simulink model "labFinal_8"  (R2018b)
settings: Solver=FixedStepDiscrete  StartTime=0.0  StopTime=20.0  FixedStep=1  RelTol=1e-3
libraries: hdlsllib x113, simulink_extras x8
(part 3 of 4)

== system labFinal_8/8-Bit_Processor/8-bit 4-1 MUX/4-1 MUX 2^6/2-1 MUX1 ==
  S : Inport  OutDataTypeStr=boolean
  I0 : Inport  Port=2  OutDataTypeStr=boolean
  I1 : Inport  Port=3  OutDataTypeStr=boolean
  Logical Operator : Logic  AllPortsSameDT=off  OutDataTypeStr=boolean
  Logical Operator1 : Logic  AllPortsSameDT=off  OutDataTypeStr=boolean
  Logical Operator2 : Logic  Operator=OR  AllPortsSameDT=off  OutDataTypeStr=boolean
  Logical Operator3 : Logic  Operator=NOT  AllPortsSameDT=off  OutDataTypeStr=boolean
  Z : Outport
  wires:
  Logical Operator2/1 -> Z/1
  Logical Operator1/1 -> Logical Operator2/2
  S/1 -> Logical Operator3/1, Logical Operator1/1
  Logical Operator/1 -> Logical Operator2/1
  I0/1 -> Logical Operator/1
  I1/1 -> Logical Operator1/2
  Logical Operator3/1 -> Logical Operator/2

== system labFinal_8/8-Bit_Processor/8-bit 4-1 MUX/4-1 MUX 2^6/2-1 MUX2 ==
  S : Inport  OutDataTypeStr=boolean
  I0 : Inport  Port=2  OutDataTypeStr=boolean
  I1 : Inport  Port=3  OutDataTypeStr=boolean
  Logical Operator : Logic  AllPortsSameDT=off  OutDataTypeStr=boolean
  Logical Operator1 : Logic  AllPortsSameDT=off  OutDataTypeStr=boolean
  Logical Operator2 : Logic  Operator=OR  AllPortsSameDT=off  OutDataTypeStr=boolean
  Logical Operator3 : Logic  Operator=NOT  AllPortsSameDT=off  OutDataTypeStr=boolean
  Z : Outport
  wires:
  Logical Operator2/1 -> Z/1
  Logical Operator1/1 -> Logical Operator2/2
  S/1 -> Logical Operator3/1, Logical Operator1/1
  Logical Operator/1 -> Logical Operator2/1
  I0/1 -> Logical Operator/1
  I1/1 -> Logical Operator1/2
  Logical Operator3/1 -> Logical Operator/2

== system labFinal_8/8-Bit_Processor/8-bit 4-1 MUX/4-1 MUX 2^6/2-1 MUX3 ==
  S : Inport  OutDataTypeStr=boolean
  I0 : Inport  Port=2  OutDataTypeStr=boolean
  I1 : Inport  Port=3  OutDataTypeStr=boolean
  Logical Operator : Logic  AllPortsSameDT=off  OutDataTypeStr=boolean
  Logical Operator1 : Logic  AllPortsSameDT=off  OutDataTypeStr=boolean
  Logical Operator2 : Logic  Operator=OR  AllPortsSameDT=off  OutDataTypeStr=boolean
  Logical Operator3 : Logic  Operator=NOT  AllPortsSameDT=off  OutDataTypeStr=boolean
  Z : Outport
  wires:
  Logical Operator2/1 -> Z/1
  Logical Operator1/1 -> Logical Operator2/2
  S/1 -> Logical Operator3/1, Logical Operator1/1
  Logical Operator/1 -> Logical Operator2/1
  I0/1 -> Logical Operator/1
  I1/1 -> Logical Operator1/2
  Logical Operator3/1 -> Logical Operator/2

== system labFinal_8/8-Bit_Processor/8-bit 4-1 MUX/4-1 MUX 2^7/2-1 MUX1 ==
  S : Inport  OutDataTypeStr=boolean
  I0 : Inport  Port=2  OutDataTypeStr=boolean
  I1 : Inport  Port=3  OutDataTypeStr=boolean
  Logical Operator : Logic  AllPortsSameDT=off  OutDataTypeStr=boolean
  Logical Operator1 : Logic  AllPortsSameDT=off  OutDataTypeStr=boolean
  Logical Operator2 : Logic  Operator=OR  AllPortsSameDT=off  OutDataTypeStr=boolean
  Logical Operator3 : Logic  Operator=NOT  AllPortsSameDT=off  OutDataTypeStr=boolean
  Z : Outport
  wires:
  Logical Operator2/1 -> Z/1
  Logical Operator1/1 -> Logical Operator2/2
  S/1 -> Logical Operator3/1, Logical Operator1/1
  Logical Operator/1 -> Logical Operator2/1
  I0/1 -> Logical Operator/1
  I1/1 -> Logical Operator1/2
  Logical Operator3/1 -> Logical Operator/2

== system labFinal_8/8-Bit_Processor/8-bit 4-1 MUX/4-1 MUX 2^7/2-1 MUX2 ==
  S : Inport  OutDataTypeStr=boolean
  I0 : Inport  Port=2  OutDataTypeStr=boolean
  I1 : Inport  Port=3  OutDataTypeStr=boolean
  Logical Operator : Logic  AllPortsSameDT=off  OutDataTypeStr=boolean
  Logical Operator1 : Logic  AllPortsSameDT=off  OutDataTypeStr=boolean
  Logical Operator2 : Logic  Operator=OR  AllPortsSameDT=off  OutDataTypeStr=boolean
  Logical Operator3 : Logic  Operator=NOT  AllPortsSameDT=off  OutDataTypeStr=boolean
  Z : Outport
  wires:
  Logical Operator2/1 -> Z/1
  Logical Operator1/1 -> Logical Operator2/2
  S/1 -> Logical Operator3/1, Logical Operator1/1
  Logical Operator/1 -> Logical Operator2/1
  I0/1 -> Logical Operator/1
  I1/1 -> Logical Operator1/2
  Logical Operator3/1 -> Logical Operator/2

== system labFinal_8/8-Bit_Processor/8-bit 4-1 MUX/4-1 MUX 2^7/2-1 MUX3 ==
  S : Inport  OutDataTypeStr=boolean
  I0 : Inport  Port=2  OutDataTypeStr=boolean
  I1 : Inport  Port=3  OutDataTypeStr=boolean
  Logical Operator : Logic  AllPortsSameDT=off  OutDataTypeStr=boolean
  Logical Operator1 : Logic  AllPortsSameDT=off  OutDataTypeStr=boolean
  Logical Operator2 : Logic  Operator=OR  AllPortsSameDT=off  OutDataTypeStr=boolean
  Logical Operator3 : Logic  Operator=NOT  AllPortsSameDT=off  OutDataTypeStr=boolean
  Z : Outport
  wires:
  Logical Operator2/1 -> Z/1
  Logical Operator1/1 -> Logical Operator2/2
  S/1 -> Logical Operator3/1, Logical Operator1/1
  Logical Operator/1 -> Logical Operator2/1
  I0/1 -> Logical Operator/1
  I1/1 -> Logical Operator1/2
  Logical Operator3/1 -> Logical Operator/2

== system labFinal_8/8-Bit_Processor/8-bit 4-1 MUX/4-1 MUX 2^8/2-1 MUX1 ==
  S : Inport  OutDataTypeStr=boolean
  I0 : Inport  Port=2  OutDataTypeStr=boolean
  I1 : Inport  Port=3  OutDataTypeStr=boolean
  Logical Operator : Logic  AllPortsSameDT=off  OutDataTypeStr=boolean
  Logical Operator1 : Logic  AllPortsSameDT=off  OutDataTypeStr=boolean
  Logical Operator2 : Logic  Operator=OR  AllPortsSameDT=off  OutDataTypeStr=boolean
  Logical Operator3 : Logic  Operator=NOT  AllPortsSameDT=off  OutDataTypeStr=boolean
  Z : Outport
  wires:
  Logical Operator2/1 -> Z/1
  Logical Operator1/1 -> Logical Operator2/2
  S/1 -> Logical Operator3/1, Logical Operator1/1
  Logical Operator/1 -> Logical Operator2/1
  I0/1 -> Logical Operator/1
  I1/1 -> Logical Operator1/2
  Logical Operator3/1 -> Logical Operator/2

== system labFinal_8/8-Bit_Processor/8-bit 4-1 MUX/4-1 MUX 2^8/2-1 MUX2 ==
  S : Inport  OutDataTypeStr=boolean
  I0 : Inport  Port=2  OutDataTypeStr=boolean
  I1 : Inport  Port=3  OutDataTypeStr=boolean
  Logical Operator : Logic  AllPortsSameDT=off  OutDataTypeStr=boolean
  Logical Operator1 : Logic  AllPortsSameDT=off  OutDataTypeStr=boolean
  Logical Operator2 : Logic  Operator=OR  AllPortsSameDT=off  OutDataTypeStr=boolean
  Logical Operator3 : Logic  Operator=NOT  AllPortsSameDT=off  OutDataTypeStr=boolean
  Z : Outport
  wires:
  Logical Operator2/1 -> Z/1
  Logical Operator1/1 -> Logical Operator2/2
  S/1 -> Logical Operator3/1, Logical Operator1/1
  Logical Operator/1 -> Logical Operator2/1
  I0/1 -> Logical Operator/1
  I1/1 -> Logical Operator1/2
  Logical Operator3/1 -> Logical Operator/2

== system labFinal_8/8-Bit_Processor/8-bit 4-1 MUX/4-1 MUX 2^8/2-1 MUX3 ==
  S : Inport  OutDataTypeStr=boolean
  I0 : Inport  Port=2  OutDataTypeStr=boolean
  I1 : Inport  Port=3  OutDataTypeStr=boolean
  Logical Operator : Logic  AllPortsSameDT=off  OutDataTypeStr=boolean
  Logical Operator1 : Logic  AllPortsSameDT=off  OutDataTypeStr=boolean
  Logical Operator2 : Logic  Operator=OR  AllPortsSameDT=off  OutDataTypeStr=boolean
  Logical Operator3 : Logic  Operator=NOT  AllPortsSameDT=off  OutDataTypeStr=boolean
  Z : Outport
  wires:
  Logical Operator2/1 -> Z/1
  Logical Operator1/1 -> Logical Operator2/2
  S/1 -> Logical Operator3/1, Logical Operator1/1
  Logical Operator/1 -> Logical Operator2/1
  I0/1 -> Logical Operator/1
  I1/1 -> Logical Operator1/2
  Logical Operator3/1 -> Logical Operator/2

== system labFinal_8/8-Bit_Processor/8-bit Adder/2^0/Half_Adder ==
  x : Inport
  y : Inport  Port=2
  Calc Carry : Logic  AllPortsSameDT=off  OutDataTypeStr=boolean
  Calc Sum : Logic  Operator=XOR  AllPortsSameDT=off  OutDataTypeStr=boolean
  Sum : Outport
  Carry : Outport  Port=2
  wires:
  Calc Carry/1 -> Carry/1
  x/1 -> Calc Carry/1, Calc Sum/1
  Calc Sum/1 -> Sum/1
  y/1 -> Calc Sum/2, Calc Carry/2

== system labFinal_8/8-Bit_Processor/8-bit Adder/2^0/Half_Adder1 ==
  x : Inport
  y : Inport  Port=2
  Calc Carry : Logic  AllPortsSameDT=off  OutDataTypeStr=boolean
  Calc Sum : Logic  Operator=XOR  AllPortsSameDT=off  OutDataTypeStr=boolean
  Sum : Outport
  Carry : Outport  Port=2
  wires:
  Calc Carry/1 -> Carry/1
  x/1 -> Calc Carry/1, Calc Sum/1
  Calc Sum/1 -> Sum/1
  y/1 -> Calc Sum/2, Calc Carry/2

== system labFinal_8/8-Bit_Processor/8-bit Adder/2^1/Half_Adder ==
  x : Inport
  y : Inport  Port=2
  Calc Carry : Logic  AllPortsSameDT=off  OutDataTypeStr=boolean
  Calc Sum : Logic  Operator=XOR  AllPortsSameDT=off  OutDataTypeStr=boolean
  Sum : Outport
  Carry : Outport  Port=2
  wires:
  Calc Carry/1 -> Carry/1
  x/1 -> Calc Carry/1, Calc Sum/1
  Calc Sum/1 -> Sum/1
  y/1 -> Calc Sum/2, Calc Carry/2

== system labFinal_8/8-Bit_Processor/8-bit Adder/2^1/Half_Adder1 ==
  x : Inport
  y : Inport  Port=2
  Calc Carry : Logic  AllPortsSameDT=off  OutDataTypeStr=boolean
  Calc Sum : Logic  Operator=XOR  AllPortsSameDT=off  OutDataTypeStr=boolean
  Sum : Outport
  Carry : Outport  Port=2
  wires:
  Calc Carry/1 -> Carry/1
  x/1 -> Calc Carry/1, Calc Sum/1
  Calc Sum/1 -> Sum/1
  y/1 -> Calc Sum/2, Calc Carry/2

== system labFinal_8/8-Bit_Processor/8-bit Adder/2^2/Half_Adder ==
  x : Inport
  y : Inport  Port=2
  Calc Carry : Logic  AllPortsSameDT=off  OutDataTypeStr=boolean
  Calc Sum : Logic  Operator=XOR  AllPortsSameDT=off  OutDataTypeStr=boolean
  Sum : Outport
  Carry : Outport  Port=2
  wires:
  Calc Carry/1 -> Carry/1
  x/1 -> Calc Carry/1, Calc Sum/1
  Calc Sum/1 -> Sum/1
  y/1 -> Calc Sum/2, Calc Carry/2

== system labFinal_8/8-Bit_Processor/8-bit Adder/2^2/Half_Adder1 ==
  x : Inport
  y : Inport  Port=2
  Calc Carry : Logic  AllPortsSameDT=off  OutDataTypeStr=boolean
  Calc Sum : Logic  Operator=XOR  AllPortsSameDT=off  OutDataTypeStr=boolean
  Sum : Outport
  Carry : Outport  Port=2
  wires:
  Calc Carry/1 -> Carry/1
  x/1 -> Calc Carry/1, Calc Sum/1
  Calc Sum/1 -> Sum/1
  y/1 -> Calc Sum/2, Calc Carry/2

== system labFinal_8/8-Bit_Processor/8-bit Adder/2^3/Half_Adder ==
  x : Inport
  y : Inport  Port=2
  Calc Carry : Logic  AllPortsSameDT=off  OutDataTypeStr=boolean
  Calc Sum : Logic  Operator=XOR  AllPortsSameDT=off  OutDataTypeStr=boolean
  Sum : Outport
  Carry : Outport  Port=2
  wires:
  Calc Carry/1 -> Carry/1
  x/1 -> Calc Carry/1, Calc Sum/1
  Calc Sum/1 -> Sum/1
  y/1 -> Calc Sum/2, Calc Carry/2

== system labFinal_8/8-Bit_Processor/8-bit Adder/2^3/Half_Adder1 ==
  x : Inport
  y : Inport  Port=2
  Calc Carry : Logic  AllPortsSameDT=off  OutDataTypeStr=boolean
  Calc Sum : Logic  Operator=XOR  AllPortsSameDT=off  OutDataTypeStr=boolean
  Sum : Outport
  Carry : Outport  Port=2
  wires:
  Calc Carry/1 -> Carry/1
  x/1 -> Calc Carry/1, Calc Sum/1
  Calc Sum/1 -> Sum/1
  y/1 -> Calc Sum/2, Calc Carry/2

== system labFinal_8/8-Bit_Processor/8-bit Adder/2^4/Half_Adder ==
  x : Inport
  y : Inport  Port=2
  Calc Carry : Logic  AllPortsSameDT=off  OutDataTypeStr=boolean
  Calc Sum : Logic  Operator=XOR  AllPortsSameDT=off  OutDataTypeStr=boolean
  Sum : Outport
  Carry : Outport  Port=2
  wires:
  Calc Carry/1 -> Carry/1
  x/1 -> Calc Carry/1, Calc Sum/1
  Calc Sum/1 -> Sum/1
  y/1 -> Calc Sum/2, Calc Carry/2

== system labFinal_8/8-Bit_Processor/8-bit Adder/2^4/Half_Adder1 ==
  x : Inport
  y : Inport  Port=2
  Calc Carry : Logic  AllPortsSameDT=off  OutDataTypeStr=boolean
  Calc Sum : Logic  Operator=XOR  AllPortsSameDT=off  OutDataTypeStr=boolean
  Sum : Outport
  Carry : Outport  Port=2
  wires:
  Calc Carry/1 -> Carry/1
  x/1 -> Calc Carry/1, Calc Sum/1
  Calc Sum/1 -> Sum/1
  y/1 -> Calc Sum/2, Calc Carry/2

== system labFinal_8/8-Bit_Processor/8-bit Adder/2^5/Half_Adder ==
  x : Inport
  y : Inport  Port=2
  Calc Carry : Logic  AllPortsSameDT=off  OutDataTypeStr=boolean
  Calc Sum : Logic  Operator=XOR  AllPortsSameDT=off  OutDataTypeStr=boolean
  Sum : Outport
  Carry : Outport  Port=2
  wires:
  Calc Carry/1 -> Carry/1
  x/1 -> Calc Carry/1, Calc Sum/1
  Calc Sum/1 -> Sum/1
  y/1 -> Calc Sum/2, Calc Carry/2

== system labFinal_8/8-Bit_Processor/8-bit Adder/2^5/Half_Adder1 ==
  x : Inport
  y : Inport  Port=2
  Calc Carry : Logic  AllPortsSameDT=off  OutDataTypeStr=boolean
  Calc Sum : Logic  Operator=XOR  AllPortsSameDT=off  OutDataTypeStr=boolean
  Sum : Outport
  Carry : Outport  Port=2
  wires:
  Calc Carry/1 -> Carry/1
  x/1 -> Calc Carry/1, Calc Sum/1
  Calc Sum/1 -> Sum/1
  y/1 -> Calc Sum/2, Calc Carry/2

== system labFinal_8/8-Bit_Processor/8-bit Adder/2^6/Half_Adder ==
  x : Inport
  y : Inport  Port=2
  Calc Carry : Logic  AllPortsSameDT=off  OutDataTypeStr=boolean
  Calc Sum : Logic  Operator=XOR  AllPortsSameDT=off  OutDataTypeStr=boolean
  Sum : Outport
  Carry : Outport  Port=2
  wires:
  Calc Carry/1 -> Carry/1
  x/1 -> Calc Carry/1, Calc Sum/1
  Calc Sum/1 -> Sum/1
  y/1 -> Calc Sum/2, Calc Carry/2

== system labFinal_8/8-Bit_Processor/8-bit Adder/2^6/Half_Adder1 ==
  x : Inport
  y : Inport  Port=2
  Calc Carry : Logic  AllPortsSameDT=off  OutDataTypeStr=boolean
  Calc Sum : Logic  Operator=XOR  AllPortsSameDT=off  OutDataTypeStr=boolean
  Sum : Outport
  Carry : Outport  Port=2
  wires:
  Calc Carry/1 -> Carry/1
  x/1 -> Calc Carry/1, Calc Sum/1
  Calc Sum/1 -> Sum/1
  y/1 -> Calc Sum/2, Calc Carry/2

== system labFinal_8/8-Bit_Processor/8-bit Adder/2^7/Half_Adder ==
  x : Inport
  y : Inport  Port=2
  Calc Carry : Logic  AllPortsSameDT=off  OutDataTypeStr=boolean
  Calc Sum : Logic  Operator=XOR  AllPortsSameDT=off  OutDataTypeStr=boolean
  Sum : Outport
  Carry : Outport  Port=2
  wires:
  Calc Carry/1 -> Carry/1
  x/1 -> Calc Carry/1, Calc Sum/1
  Calc Sum/1 -> Sum/1
  y/1 -> Calc Sum/2, Calc Carry/2

== system labFinal_8/8-Bit_Processor/8-bit Adder/2^7/Half_Adder1 ==
  x : Inport
  y : Inport  Port=2
  Calc Carry : Logic  AllPortsSameDT=off  OutDataTypeStr=boolean
  Calc Sum : Logic  Operator=XOR  AllPortsSameDT=off  OutDataTypeStr=boolean
  Sum : Outport
  Carry : Outport  Port=2
  wires:
  Calc Carry/1 -> Carry/1
  x/1 -> Calc Carry/1, Calc Sum/1
  Calc Sum/1 -> Sum/1
  y/1 -> Calc Sum/2, Calc Carry/2

== system labFinal_8/8-Bit_Processor/8-bit Multiply/2^1/Half_Adder ==
  x : Inport
  y : Inport  Port=2
  Calc Carry : Logic  AllPortsSameDT=off  OutDataTypeStr=boolean
  Calc Sum : Logic  Operator=XOR  AllPortsSameDT=off  OutDataTypeStr=boolean
  Sum : Outport
  Carry : Outport  Port=2
  wires:
  Calc Carry/1 -> Carry/1
  x/1 -> Calc Carry/1, Calc Sum/1
  Calc Sum/1 -> Sum/1
  y/1 -> Calc Sum/2, Calc Carry/2

== system labFinal_8/8-Bit_Processor/8-bit Multiply/2^1/Half_Adder1 ==
  x : Inport
  y : Inport  Port=2
  Calc Carry : Logic  AllPortsSameDT=off  OutDataTypeStr=boolean
  Calc Sum : Logic  Operator=XOR  AllPortsSameDT=off  OutDataTypeStr=boolean
  Sum : Outport
  Carry : Outport  Port=2
  wires:
  Calc Carry/1 -> Carry/1
  x/1 -> Calc Carry/1, Calc Sum/1
  Calc Sum/1 -> Sum/1
  y/1 -> Calc Sum/2, Calc Carry/2

== system labFinal_8/8-Bit_Processor/8-bit Multiply/2^10/Half_Adder ==
  x : Inport
  y : Inport  Port=2
  Calc Carry : Logic  AllPortsSameDT=off  OutDataTypeStr=boolean
  Calc Sum : Logic  Operator=XOR  AllPortsSameDT=off  OutDataTypeStr=boolean
  Sum : Outport
  Carry : Outport  Port=2
  wires:
  Calc Carry/1 -> Carry/1
  x/1 -> Calc Carry/1, Calc Sum/1
  Calc Sum/1 -> Sum/1
  y/1 -> Calc Sum/2, Calc Carry/2

== system labFinal_8/8-Bit_Processor/8-bit Multiply/2^10/Half_Adder1 ==
  x : Inport
  y : Inport  Port=2
  Calc Carry : Logic  AllPortsSameDT=off  OutDataTypeStr=boolean
  Calc Sum : Logic  Operator=XOR  AllPortsSameDT=off  OutDataTypeStr=boolean
  Sum : Outport
  Carry : Outport  Port=2
  wires:
  Calc Carry/1 -> Carry/1
  x/1 -> Calc Carry/1, Calc Sum/1
  Calc Sum/1 -> Sum/1
  y/1 -> Calc Sum/2, Calc Carry/2

== system labFinal_8/8-Bit_Processor/8-bit Multiply/2^11/Half_Adder ==
  x : Inport
  y : Inport  Port=2
  Calc Carry : Logic  AllPortsSameDT=off  OutDataTypeStr=boolean
  Calc Sum : Logic  Operator=XOR  AllPortsSameDT=off  OutDataTypeStr=boolean
  Sum : Outport
  Carry : Outport  Port=2
  wires:
  Calc Carry/1 -> Carry/1
  x/1 -> Calc Carry/1, Calc Sum/1
  Calc Sum/1 -> Sum/1
  y/1 -> Calc Sum/2, Calc Carry/2

== system labFinal_8/8-Bit_Processor/8-bit Multiply/2^11/Half_Adder1 ==
  x : Inport
  y : Inport  Port=2
  Calc Carry : Logic  AllPortsSameDT=off  OutDataTypeStr=boolean
  Calc Sum : Logic  Operator=XOR  AllPortsSameDT=off  OutDataTypeStr=boolean
  Sum : Outport
  Carry : Outport  Port=2
  wires:
  Calc Carry/1 -> Carry/1
  x/1 -> Calc Carry/1, Calc Sum/1
  Calc Sum/1 -> Sum/1
  y/1 -> Calc Sum/2, Calc Carry/2

== system labFinal_8/8-Bit_Processor/8-bit Multiply/2^12/Half_Adder ==
  x : Inport
  y : Inport  Port=2
  Calc Carry : Logic  AllPortsSameDT=off  OutDataTypeStr=boolean
  Calc Sum : Logic  Operator=XOR  AllPortsSameDT=off  OutDataTypeStr=boolean
  Sum : Outport
  Carry : Outport  Port=2
  wires:
  Calc Carry/1 -> Carry/1
  x/1 -> Calc Carry/1, Calc Sum/1
  Calc Sum/1 -> Sum/1
  y/1 -> Calc Sum/2, Calc Carry/2

== system labFinal_8/8-Bit_Processor/8-bit Multiply/2^12/Half_Adder1 ==
  x : Inport
  y : Inport  Port=2
  Calc Carry : Logic  AllPortsSameDT=off  OutDataTypeStr=boolean
  Calc Sum : Logic  Operator=XOR  AllPortsSameDT=off  OutDataTypeStr=boolean
  Sum : Outport
  Carry : Outport  Port=2
  wires:
  Calc Carry/1 -> Carry/1
  x/1 -> Calc Carry/1, Calc Sum/1
  Calc Sum/1 -> Sum/1
  y/1 -> Calc Sum/2, Calc Carry/2

== system labFinal_8/8-Bit_Processor/8-bit Multiply/2^13/Half_Adder ==
  x : Inport
  y : Inport  Port=2
  Calc Carry : Logic  AllPortsSameDT=off  OutDataTypeStr=boolean
  Calc Sum : Logic  Operator=XOR  AllPortsSameDT=off  OutDataTypeStr=boolean
  Sum : Outport
  Carry : Outport  Port=2
  wires:
  Calc Carry/1 -> Carry/1
  x/1 -> Calc Carry/1, Calc Sum/1
  Calc Sum/1 -> Sum/1
  y/1 -> Calc Sum/2, Calc Carry/2

== system labFinal_8/8-Bit_Processor/8-bit Multiply/2^13/Half_Adder1 ==
  x : Inport
  y : Inport  Port=2
  Calc Carry : Logic  AllPortsSameDT=off  OutDataTypeStr=boolean
  Calc Sum : Logic  Operator=XOR  AllPortsSameDT=off  OutDataTypeStr=boolean
  Sum : Outport
  Carry : Outport  Port=2
  wires:
  Calc Carry/1 -> Carry/1
  x/1 -> Calc Carry/1, Calc Sum/1
  Calc Sum/1 -> Sum/1
  y/1 -> Calc Sum/2, Calc Carry/2

== system labFinal_8/8-Bit_Processor/8-bit Multiply/2^14/Half_Adder ==
  x : Inport
  y : Inport  Port=2
  Calc Carry : Logic  AllPortsSameDT=off  OutDataTypeStr=boolean
  Calc Sum : Logic  Operator=XOR  AllPortsSameDT=off  OutDataTypeStr=boolean
  Sum : Outport
  Carry : Outport  Port=2
  wires:
  Calc Carry/1 -> Carry/1
  x/1 -> Calc Carry/1, Calc Sum/1
  Calc Sum/1 -> Sum/1
  y/1 -> Calc Sum/2, Calc Carry/2

== system labFinal_8/8-Bit_Processor/8-bit Multiply/2^14/Half_Adder1 ==
  x : Inport
  y : Inport  Port=2
  Calc Carry : Logic  AllPortsSameDT=off  OutDataTypeStr=boolean
  Calc Sum : Logic  Operator=XOR  AllPortsSameDT=off  OutDataTypeStr=boolean
  Sum : Outport
  Carry : Outport  Port=2
  wires:
  Calc Carry/1 -> Carry/1
  x/1 -> Calc Carry/1, Calc Sum/1
  Calc Sum/1 -> Sum/1
  y/1 -> Calc Sum/2, Calc Carry/2

== system labFinal_8/8-Bit_Processor/8-bit Multiply/2^15/Half_Adder ==
  x : Inport
  y : Inport  Port=2
  Calc Carry : Logic  AllPortsSameDT=off  OutDataTypeStr=boolean
  Calc Sum : Logic  Operator=XOR  AllPortsSameDT=off  OutDataTypeStr=boolean
  Sum : Outport
  Carry : Outport  Port=2
  wires:
  Calc Carry/1 -> Carry/1
  x/1 -> Calc Carry/1, Calc Sum/1
  Calc Sum/1 -> Sum/1
  y/1 -> Calc Sum/2, Calc Carry/2

== system labFinal_8/8-Bit_Processor/8-bit Multiply/2^15/Half_Adder1 ==
  x : Inport
  y : Inport  Port=2
  Calc Carry : Logic  AllPortsSameDT=off  OutDataTypeStr=boolean
  Calc Sum : Logic  Operator=XOR  AllPortsSameDT=off  OutDataTypeStr=boolean
  Sum : Outport
  Carry : Outport  Port=2
  wires:
  Calc Carry/1 -> Carry/1
  x/1 -> Calc Carry/1, Calc Sum/1
  Calc Sum/1 -> Sum/1
  y/1 -> Calc Sum/2, Calc Carry/2

== system labFinal_8/8-Bit_Processor/8-bit Multiply/2^16/Half_Adder ==
  x : Inport
  y : Inport  Port=2
  Calc Carry : Logic  AllPortsSameDT=off  OutDataTypeStr=boolean
  Calc Sum : Logic  Operator=XOR  AllPortsSameDT=off  OutDataTypeStr=boolean
  Sum : Outport
  Carry : Outport  Port=2
  wires:
  Calc Carry/1 -> Carry/1
  x/1 -> Calc Carry/1, Calc Sum/1
  Calc Sum/1 -> Sum/1
  y/1 -> Calc Sum/2, Calc Carry/2

== system labFinal_8/8-Bit_Processor/8-bit Multiply/2^16/Half_Adder1 ==
  x : Inport
  y : Inport  Port=2
  Calc Carry : Logic  AllPortsSameDT=off  OutDataTypeStr=boolean
  Calc Sum : Logic  Operator=XOR  AllPortsSameDT=off  OutDataTypeStr=boolean
  Sum : Outport
  Carry : Outport  Port=2
  wires:
  Calc Carry/1 -> Carry/1
  x/1 -> Calc Carry/1, Calc Sum/1
  Calc Sum/1 -> Sum/1
  y/1 -> Calc Sum/2, Calc Carry/2

== system labFinal_8/8-Bit_Processor/8-bit Multiply/2^17/Half_Adder ==
  x : Inport
  y : Inport  Port=2
  Calc Carry : Logic  AllPortsSameDT=off  OutDataTypeStr=boolean
  Calc Sum : Logic  Operator=XOR  AllPortsSameDT=off  OutDataTypeStr=boolean
  Sum : Outport
  Carry : Outport  Port=2
  wires:
  Calc Carry/1 -> Carry/1
  x/1 -> Calc Carry/1, Calc Sum/1
  Calc Sum/1 -> Sum/1
  y/1 -> Calc Sum/2, Calc Carry/2

== system labFinal_8/8-Bit_Processor/8-bit Multiply/2^17/Half_Adder1 ==
  x : Inport
  y : Inport  Port=2
  Calc Carry : Logic  AllPortsSameDT=off  OutDataTypeStr=boolean
  Calc Sum : Logic  Operator=XOR  AllPortsSameDT=off  OutDataTypeStr=boolean
  Sum : Outport
  Carry : Outport  Port=2
  wires:
  Calc Carry/1 -> Carry/1
  x/1 -> Calc Carry/1, Calc Sum/1
  Calc Sum/1 -> Sum/1
  y/1 -> Calc Sum/2, Calc Carry/2

== system labFinal_8/8-Bit_Processor/8-bit Multiply/2^18/Half_Adder ==
  x : Inport
  y : Inport  Port=2
  Calc Carry : Logic  AllPortsSameDT=off  OutDataTypeStr=boolean
  Calc Sum : Logic  Operator=XOR  AllPortsSameDT=off  OutDataTypeStr=boolean
  Sum : Outport
  Carry : Outport  Port=2
  wires:
  Calc Carry/1 -> Carry/1
  x/1 -> Calc Carry/1, Calc Sum/1
  Calc Sum/1 -> Sum/1
  y/1 -> Calc Sum/2, Calc Carry/2

== system labFinal_8/8-Bit_Processor/8-bit Multiply/2^18/Half_Adder1 ==
  x : Inport
  y : Inport  Port=2
  Calc Carry : Logic  AllPortsSameDT=off  OutDataTypeStr=boolean
  Calc Sum : Logic  Operator=XOR  AllPortsSameDT=off  OutDataTypeStr=boolean
  Sum : Outport
  Carry : Outport  Port=2
  wires:
  Calc Carry/1 -> Carry/1
  x/1 -> Calc Carry/1, Calc Sum/1
  Calc Sum/1 -> Sum/1
  y/1 -> Calc Sum/2, Calc Carry/2

== system labFinal_8/8-Bit_Processor/8-bit Multiply/2^19/Half_Adder ==
  x : Inport
  y : Inport  Port=2
  Calc Carry : Logic  AllPortsSameDT=off  OutDataTypeStr=boolean
  Calc Sum : Logic  Operator=XOR  AllPortsSameDT=off  OutDataTypeStr=boolean
  Sum : Outport
  Carry : Outport  Port=2
  wires:
  Calc Carry/1 -> Carry/1
  x/1 -> Calc Carry/1, Calc Sum/1
  Calc Sum/1 -> Sum/1
  y/1 -> Calc Sum/2, Calc Carry/2

== system labFinal_8/8-Bit_Processor/8-bit Multiply/2^19/Half_Adder1 ==
  x : Inport
  y : Inport  Port=2
  Calc Carry : Logic  AllPortsSameDT=off  OutDataTypeStr=boolean
  Calc Sum : Logic  Operator=XOR  AllPortsSameDT=off  OutDataTypeStr=boolean
  Sum : Outport
  Carry : Outport  Port=2
  wires:
  Calc Carry/1 -> Carry/1
  x/1 -> Calc Carry/1, Calc Sum/1
  Calc Sum/1 -> Sum/1
  y/1 -> Calc Sum/2, Calc Carry/2

== system labFinal_8/8-Bit_Processor/8-bit Multiply/2^2/Half_Adder ==
  x : Inport
  y : Inport  Port=2
  Calc Carry : Logic  AllPortsSameDT=off  OutDataTypeStr=boolean
  Calc Sum : Logic  Operator=XOR  AllPortsSameDT=off  OutDataTypeStr=boolean
  Sum : Outport
  Carry : Outport  Port=2
  wires:
  Calc Carry/1 -> Carry/1
  x/1 -> Calc Carry/1, Calc Sum/1
  Calc Sum/1 -> Sum/1
  y/1 -> Calc Sum/2, Calc Carry/2

== system labFinal_8/8-Bit_Processor/8-bit Multiply/2^2/Half_Adder1 ==
  x : Inport
  y : Inport  Port=2
  Calc Carry : Logic  AllPortsSameDT=off  OutDataTypeStr=boolean
  Calc Sum : Logic  Operator=XOR  AllPortsSameDT=off  OutDataTypeStr=boolean
  Sum : Outport
  Carry : Outport  Port=2
  wires:
  Calc Carry/1 -> Carry/1
  x/1 -> Calc Carry/1, Calc Sum/1
  Calc Sum/1 -> Sum/1
  y/1 -> Calc Sum/2, Calc Carry/2

== system labFinal_8/8-Bit_Processor/8-bit Multiply/2^20/Half_Adder ==
  x : Inport
  y : Inport  Port=2
  Calc Carry : Logic  AllPortsSameDT=off  OutDataTypeStr=boolean
  Calc Sum : Logic  Operator=XOR  AllPortsSameDT=off  OutDataTypeStr=boolean
  Sum : Outport
  Carry : Outport  Port=2
  wires:
  Calc Carry/1 -> Carry/1
  x/1 -> Calc Carry/1, Calc Sum/1
  Calc Sum/1 -> Sum/1
  y/1 -> Calc Sum/2, Calc Carry/2

== system labFinal_8/8-Bit_Processor/8-bit Multiply/2^20/Half_Adder1 ==
  x : Inport
  y : Inport  Port=2
  Calc Carry : Logic  AllPortsSameDT=off  OutDataTypeStr=boolean
  Calc Sum : Logic  Operator=XOR  AllPortsSameDT=off  OutDataTypeStr=boolean
  Sum : Outport
  Carry : Outport  Port=2
  wires:
  Calc Carry/1 -> Carry/1
  x/1 -> Calc Carry/1, Calc Sum/1
  Calc Sum/1 -> Sum/1
  y/1 -> Calc Sum/2, Calc Carry/2

== system labFinal_8/8-Bit_Processor/8-bit Multiply/2^21/Half_Adder ==
  x : Inport
  y : Inport  Port=2
  Calc Carry : Logic  AllPortsSameDT=off  OutDataTypeStr=boolean
  Calc Sum : Logic  Operator=XOR  AllPortsSameDT=off  OutDataTypeStr=boolean
  Sum : Outport
  Carry : Outport  Port=2
  wires:
  Calc Carry/1 -> Carry/1
  x/1 -> Calc Carry/1, Calc Sum/1
  Calc Sum/1 -> Sum/1
  y/1 -> Calc Sum/2, Calc Carry/2

== system labFinal_8/8-Bit_Processor/8-bit Multiply/2^21/Half_Adder1 ==
  x : Inport
  y : Inport  Port=2
  Calc Carry : Logic  AllPortsSameDT=off  OutDataTypeStr=boolean
  Calc Sum : Logic  Operator=XOR  AllPortsSameDT=off  OutDataTypeStr=boolean
  Sum : Outport
  Carry : Outport  Port=2
  wires:
  Calc Carry/1 -> Carry/1
  x/1 -> Calc Carry/1, Calc Sum/1
  Calc Sum/1 -> Sum/1
  y/1 -> Calc Sum/2, Calc Carry/2

== system labFinal_8/8-Bit_Processor/8-bit Multiply/2^22/Half_Adder ==
  x : Inport
  y : Inport  Port=2
  Calc Carry : Logic  AllPortsSameDT=off  OutDataTypeStr=boolean
  Calc Sum : Logic  Operator=XOR  AllPortsSameDT=off  OutDataTypeStr=boolean
  Sum : Outport
  Carry : Outport  Port=2
  wires:
  Calc Carry/1 -> Carry/1
  x/1 -> Calc Carry/1, Calc Sum/1
  Calc Sum/1 -> Sum/1
  y/1 -> Calc Sum/2, Calc Carry/2

== system labFinal_8/8-Bit_Processor/8-bit Multiply/2^22/Half_Adder1 ==
  x : Inport
  y : Inport  Port=2
  Calc Carry : Logic  AllPortsSameDT=off  OutDataTypeStr=boolean
  Calc Sum : Logic  Operator=XOR  AllPortsSameDT=off  OutDataTypeStr=boolean
  Sum : Outport
  Carry : Outport  Port=2
  wires:
  Calc Carry/1 -> Carry/1
  x/1 -> Calc Carry/1, Calc Sum/1
  Calc Sum/1 -> Sum/1
  y/1 -> Calc Sum/2, Calc Carry/2

== system labFinal_8/8-Bit_Processor/8-bit Multiply/2^23/Half_Adder ==
  x : Inport
  y : Inport  Port=2
  Calc Carry : Logic  AllPortsSameDT=off  OutDataTypeStr=boolean
  Calc Sum : Logic  Operator=XOR  AllPortsSameDT=off  OutDataTypeStr=boolean
  Sum : Outport
  Carry : Outport  Port=2
  wires:
  Calc Carry/1 -> Carry/1
  x/1 -> Calc Carry/1, Calc Sum/1
  Calc Sum/1 -> Sum/1
  y/1 -> Calc Sum/2, Calc Carry/2

== system labFinal_8/8-Bit_Processor/8-bit Multiply/2^23/Half_Adder1 ==
  x : Inport
  y : Inport  Port=2
  Calc Carry : Logic  AllPortsSameDT=off  OutDataTypeStr=boolean
  Calc Sum : Logic  Operator=XOR  AllPortsSameDT=off  OutDataTypeStr=boolean
  Sum : Outport
  Carry : Outport  Port=2
  wires:
  Calc Carry/1 -> Carry/1
  x/1 -> Calc Carry/1, Calc Sum/1
  Calc Sum/1 -> Sum/1
  y/1 -> Calc Sum/2, Calc Carry/2

== system labFinal_8/8-Bit_Processor/8-bit Multiply/2^24/Half_Adder ==
  x : Inport
  y : Inport  Port=2
  Calc Carry : Logic  AllPortsSameDT=off  OutDataTypeStr=boolean
  Calc Sum : Logic  Operator=XOR  AllPortsSameDT=off  OutDataTypeStr=boolean
  Sum : Outport
  Carry : Outport  Port=2
  wires:
  Calc Carry/1 -> Carry/1
  x/1 -> Calc Carry/1, Calc Sum/1
  Calc Sum/1 -> Sum/1
  y/1 -> Calc Sum/2, Calc Carry/2

== system labFinal_8/8-Bit_Processor/8-bit Multiply/2^24/Half_Adder1 ==
  x : Inport
  y : Inport  Port=2
  Calc Carry : Logic  AllPortsSameDT=off  OutDataTypeStr=boolean
  Calc Sum : Logic  Operator=XOR  AllPortsSameDT=off  OutDataTypeStr=boolean
  Sum : Outport
  Carry : Outport  Port=2
  wires:
  Calc Carry/1 -> Carry/1
  x/1 -> Calc Carry/1, Calc Sum/1
  Calc Sum/1 -> Sum/1
  y/1 -> Calc Sum/2, Calc Carry/2

== system labFinal_8/8-Bit_Processor/8-bit Multiply/2^25/Half_Adder ==
  x : Inport
  y : Inport  Port=2
  Calc Carry : Logic  AllPortsSameDT=off  OutDataTypeStr=boolean
  Calc Sum : Logic  Operator=XOR  AllPortsSameDT=off  OutDataTypeStr=boolean
  Sum : Outport
  Carry : Outport  Port=2
  wires:
  Calc Carry/1 -> Carry/1
  x/1 -> Calc Carry/1, Calc Sum/1
  Calc Sum/1 -> Sum/1
  y/1 -> Calc Sum/2, Calc Carry/2

== system labFinal_8/8-Bit_Processor/8-bit Multiply/2^25/Half_Adder1 ==
  x : Inport
  y : Inport  Port=2
  Calc Carry : Logic  AllPortsSameDT=off  OutDataTypeStr=boolean
  Calc Sum : Logic  Operator=XOR  AllPortsSameDT=off  OutDataTypeStr=boolean
  Sum : Outport
  Carry : Outport  Port=2
  wires:
  Calc Carry/1 -> Carry/1
  x/1 -> Calc Carry/1, Calc Sum/1
  Calc Sum/1 -> Sum/1
  y/1 -> Calc Sum/2, Calc Carry/2

== system labFinal_8/8-Bit_Processor/8-bit Multiply/2^26/Half_Adder ==
  x : Inport
  y : Inport  Port=2
  Calc Carry : Logic  AllPortsSameDT=off  OutDataTypeStr=boolean
  Calc Sum : Logic  Operator=XOR  AllPortsSameDT=off  OutDataTypeStr=boolean
  Sum : Outport
  Carry : Outport  Port=2
  wires:
  Calc Carry/1 -> Carry/1
  x/1 -> Calc Carry/1, Calc Sum/1
  Calc Sum/1 -> Sum/1
  y/1 -> Calc Sum/2, Calc Carry/2

== system labFinal_8/8-Bit_Processor/8-bit Multiply/2^26/Half_Adder1 ==
  x : Inport
  y : Inport  Port=2
  Calc Carry : Logic  AllPortsSameDT=off  OutDataTypeStr=boolean
  Calc Sum : Logic  Operator=XOR  AllPortsSameDT=off  OutDataTypeStr=boolean
  Sum : Outport
  Carry : Outport  Port=2
  wires:
  Calc Carry/1 -> Carry/1
  x/1 -> Calc Carry/1, Calc Sum/1
  Calc Sum/1 -> Sum/1
  y/1 -> Calc Sum/2, Calc Carry/2

== system labFinal_8/8-Bit_Processor/8-bit Multiply/2^27/Half_Adder ==
  x : Inport
  y : Inport  Port=2
  Calc Carry : Logic  AllPortsSameDT=off  OutDataTypeStr=boolean
  Calc Sum : Logic  Operator=XOR  AllPortsSameDT=off  OutDataTypeStr=boolean
  Sum : Outport
  Carry : Outport  Port=2
  wires:
  Calc Carry/1 -> Carry/1
  x/1 -> Calc Carry/1, Calc Sum/1
  Calc Sum/1 -> Sum/1
  y/1 -> Calc Sum/2, Calc Carry/2

== system labFinal_8/8-Bit_Processor/8-bit Multiply/2^27/Half_Adder1 ==
  x : Inport
  y : Inport  Port=2
  Calc Carry : Logic  AllPortsSameDT=off  OutDataTypeStr=boolean
  Calc Sum : Logic  Operator=XOR  AllPortsSameDT=off  OutDataTypeStr=boolean
  Sum : Outport
  Carry : Outport  Port=2
  wires:
  Calc Carry/1 -> Carry/1
  x/1 -> Calc Carry/1, Calc Sum/1
  Calc Sum/1 -> Sum/1
  y/1 -> Calc Sum/2, Calc Carry/2

== system labFinal_8/8-Bit_Processor/8-bit Multiply/2^28/Half_Adder ==
  x : Inport
  y : Inport  Port=2
  Calc Carry : Logic  AllPortsSameDT=off  OutDataTypeStr=boolean
  Calc Sum : Logic  Operator=XOR  AllPortsSameDT=off  OutDataTypeStr=boolean
  Sum : Outport
  Carry : Outport  Port=2
  wires:
  Calc Carry/1 -> Carry/1
  x/1 -> Calc Carry/1, Calc Sum/1
  Calc Sum/1 -> Sum/1
  y/1 -> Calc Sum/2, Calc Carry/2

== system labFinal_8/8-Bit_Processor/8-bit Multiply/2^28/Half_Adder1 ==
  x : Inport
  y : Inport  Port=2
  Calc Carry : Logic  AllPortsSameDT=off  OutDataTypeStr=boolean
  Calc Sum : Logic  Operator=XOR  AllPortsSameDT=off  OutDataTypeStr=boolean
  Sum : Outport
  Carry : Outport  Port=2
  wires:
  Calc Carry/1 -> Carry/1
  x/1 -> Calc Carry/1, Calc Sum/1
  Calc Sum/1 -> Sum/1
  y/1 -> Calc Sum/2, Calc Carry/2

== system labFinal_8/8-Bit_Processor/8-bit Multiply/2^29/Half_Adder ==
  x : Inport
  y : Inport  Port=2
  Calc Carry : Logic  AllPortsSameDT=off  OutDataTypeStr=boolean
  Calc Sum : Logic  Operator=XOR  AllPortsSameDT=off  OutDataTypeStr=boolean
  Sum : Outport
  Carry : Outport  Port=2
  wires:
  Calc Carry/1 -> Carry/1
  x/1 -> Calc Carry/1, Calc Sum/1
  Calc Sum/1 -> Sum/1
  y/1 -> Calc Sum/2, Calc Carry/2

== system labFinal_8/8-Bit_Processor/8-bit Multiply/2^29/Half_Adder1 ==
  x : Inport
  y : Inport  Port=2
  Calc Carry : Logic  AllPortsSameDT=off  OutDataTypeStr=boolean
  Calc Sum : Logic  Operator=XOR  AllPortsSameDT=off  OutDataTypeStr=boolean
  Sum : Outport
  Carry : Outport  Port=2
  wires:
  Calc Carry/1 -> Carry/1
  x/1 -> Calc Carry/1, Calc Sum/1
  Calc Sum/1 -> Sum/1
  y/1 -> Calc Sum/2, Calc Carry/2

== system labFinal_8/8-Bit_Processor/8-bit Multiply/2^3/Half_Adder ==
  x : Inport
  y : Inport  Port=2
  Calc Carry : Logic  AllPortsSameDT=off  OutDataTypeStr=boolean
  Calc Sum : Logic  Operator=XOR  AllPortsSameDT=off  OutDataTypeStr=boolean
  Sum : Outport
  Carry : Outport  Port=2
  wires:
  Calc Carry/1 -> Carry/1
  x/1 -> Calc Carry/1, Calc Sum/1
  Calc Sum/1 -> Sum/1
  y/1 -> Calc Sum/2, Calc Carry/2

== system labFinal_8/8-Bit_Processor/8-bit Multiply/2^3/Half_Adder1 ==
  x : Inport
  y : Inport  Port=2
  Calc Carry : Logic  AllPortsSameDT=off  OutDataTypeStr=boolean
  Calc Sum : Logic  Operator=XOR  AllPortsSameDT=off  OutDataTypeStr=boolean
  Sum : Outport
  Carry : Outport  Port=2
  wires:
  Calc Carry/1 -> Carry/1
  x/1 -> Calc Carry/1, Calc Sum/1
  Calc Sum/1 -> Sum/1
  y/1 -> Calc Sum/2, Calc Carry/2

== system labFinal_8/8-Bit_Processor/8-bit Multiply/2^30/Half_Adder ==
  x : Inport
  y : Inport  Port=2
  Calc Carry : Logic  AllPortsSameDT=off  OutDataTypeStr=boolean
  Calc Sum : Logic  Operator=XOR  AllPortsSameDT=off  OutDataTypeStr=boolean
  Sum : Outport
  Carry : Outport  Port=2
  wires:
  Calc Carry/1 -> Carry/1
  x/1 -> Calc Carry/1, Calc Sum/1
  Calc Sum/1 -> Sum/1
  y/1 -> Calc Sum/2, Calc Carry/2

== system labFinal_8/8-Bit_Processor/8-bit Multiply/2^30/Half_Adder1 ==
  x : Inport
  y : Inport  Port=2
  Calc Carry : Logic  AllPortsSameDT=off  OutDataTypeStr=boolean
  Calc Sum : Logic  Operator=XOR  AllPortsSameDT=off  OutDataTypeStr=boolean
  Sum : Outport
  Carry : Outport  Port=2
  wires:
  Calc Carry/1 -> Carry/1
  x/1 -> Calc Carry/1, Calc Sum/1
  Calc Sum/1 -> Sum/1
  y/1 -> Calc Sum/2, Calc Carry/2

== system labFinal_8/8-Bit_Processor/8-bit Multiply/2^31/Half_Adder ==
  x : Inport
  y : Inport  Port=2
  Calc Carry : Logic  AllPortsSameDT=off  OutDataTypeStr=boolean
  Calc Sum : Logic  Operator=XOR  AllPortsSameDT=off  OutDataTypeStr=boolean
  Sum : Outport
  Carry : Outport  Port=2
  wires:
  Calc Carry/1 -> Carry/1
  x/1 -> Calc Carry/1, Calc Sum/1
  Calc Sum/1 -> Sum/1
  y/1 -> Calc Sum/2, Calc Carry/2

== system labFinal_8/8-Bit_Processor/8-bit Multiply/2^31/Half_Adder1 ==
  x : Inport
  y : Inport  Port=2
  Calc Carry : Logic  AllPortsSameDT=off  OutDataTypeStr=boolean
  Calc Sum : Logic  Operator=XOR  AllPortsSameDT=off  OutDataTypeStr=boolean
  Sum : Outport
  Carry : Outport  Port=2
  wires:
  Calc Carry/1 -> Carry/1
  x/1 -> Calc Carry/1, Calc Sum/1
  Calc Sum/1 -> Sum/1
  y/1 -> Calc Sum/2, Calc Carry/2

== system labFinal_8/8-Bit_Processor/8-bit Multiply/2^32/Half_Adder ==
  x : Inport
  y : Inport  Port=2
  Calc Carry : Logic  AllPortsSameDT=off  OutDataTypeStr=boolean
  Calc Sum : Logic  Operator=XOR  AllPortsSameDT=off  OutDataTypeStr=boolean
  Sum : Outport
  Carry : Outport  Port=2
  wires:
  Calc Carry/1 -> Carry/1
  x/1 -> Calc Carry/1, Calc Sum/1
  Calc Sum/1 -> Sum/1
  y/1 -> Calc Sum/2, Calc Carry/2

== system labFinal_8/8-Bit_Processor/8-bit Multiply/2^32/Half_Adder1 ==
  x : Inport
  y : Inport  Port=2
  Calc Carry : Logic  AllPortsSameDT=off  OutDataTypeStr=boolean
  Calc Sum : Logic  Operator=XOR  AllPortsSameDT=off  OutDataTypeStr=boolean
  Sum : Outport
  Carry : Outport  Port=2
  wires:
  Calc Carry/1 -> Carry/1
  x/1 -> Calc Carry/1, Calc Sum/1
  Calc Sum/1 -> Sum/1
  y/1 -> Calc Sum/2, Calc Carry/2

== system labFinal_8/8-Bit_Processor/8-bit Multiply/2^33/Half_Adder ==
  x : Inport
  y : Inport  Port=2
  Calc Carry : Logic  AllPortsSameDT=off  OutDataTypeStr=boolean
  Calc Sum : Logic  Operator=XOR  AllPortsSameDT=off  OutDataTypeStr=boolean
  Sum : Outport
  Carry : Outport  Port=2
  wires:
  Calc Carry/1 -> Carry/1
  x/1 -> Calc Carry/1, Calc Sum/1
  Calc Sum/1 -> Sum/1
  y/1 -> Calc Sum/2, Calc Carry/2

== system labFinal_8/8-Bit_Processor/8-bit Multiply/2^33/Half_Adder1 ==
  x : Inport
  y : Inport  Port=2
  Calc Carry : Logic  AllPortsSameDT=off  OutDataTypeStr=boolean
  Calc Sum : Logic  Operator=XOR  AllPortsSameDT=off  OutDataTypeStr=boolean
  Sum : Outport
  Carry : Outport  Port=2
  wires:
  Calc Carry/1 -> Carry/1
  x/1 -> Calc Carry/1, Calc Sum/1
  Calc Sum/1 -> Sum/1
  y/1 -> Calc Sum/2, Calc Carry/2

== system labFinal_8/8-Bit_Processor/8-bit Multiply/2^34/Half_Adder ==
  x : Inport
  y : Inport  Port=2
  Calc Carry : Logic  AllPortsSameDT=off  OutDataTypeStr=boolean
  Calc Sum : Logic  Operator=XOR  AllPortsSameDT=off  OutDataTypeStr=boolean
  Sum : Outport
  Carry : Outport  Port=2
  wires:
  Calc Carry/1 -> Carry/1
  x/1 -> Calc Carry/1, Calc Sum/1
  Calc Sum/1 -> Sum/1
  y/1 -> Calc Sum/2, Calc Carry/2

== system labFinal_8/8-Bit_Processor/8-bit Multiply/2^34/Half_Adder1 ==
  x : Inport
  y : Inport  Port=2
  Calc Carry : Logic  AllPortsSameDT=off  OutDataTypeStr=boolean
  Calc Sum : Logic  Operator=XOR  AllPortsSameDT=off  OutDataTypeStr=boolean
  Sum : Outport
  Carry : Outport  Port=2
  wires:
  Calc Carry/1 -> Carry/1
  x/1 -> Calc Carry/1, Calc Sum/1
  Calc Sum/1 -> Sum/1
  y/1 -> Calc Sum/2, Calc Carry/2

== system labFinal_8/8-Bit_Processor/8-bit Multiply/2^35/Half_Adder ==
  x : Inport
  y : Inport  Port=2
  Calc Carry : Logic  AllPortsSameDT=off  OutDataTypeStr=boolean
  Calc Sum : Logic  Operator=XOR  AllPortsSameDT=off  OutDataTypeStr=boolean
  Sum : Outport
  Carry : Outport  Port=2
  wires:
  Calc Carry/1 -> Carry/1
  x/1 -> Calc Carry/1, Calc Sum/1
  Calc Sum/1 -> Sum/1
  y/1 -> Calc Sum/2, Calc Carry/2

== system labFinal_8/8-Bit_Processor/8-bit Multiply/2^35/Half_Adder1 ==
  x : Inport
  y : Inport  Port=2
  Calc Carry : Logic  AllPortsSameDT=off  OutDataTypeStr=boolean
  Calc Sum : Logic  Operator=XOR  AllPortsSameDT=off  OutDataTypeStr=boolean
  Sum : Outport
  Carry : Outport  Port=2
  wires:
  Calc Carry/1 -> Carry/1
  x/1 -> Calc Carry/1, Calc Sum/1
  Calc Sum/1 -> Sum/1
  y/1 -> Calc Sum/2, Calc Carry/2

== system labFinal_8/8-Bit_Processor/8-bit Multiply/2^36/Half_Adder ==
  x : Inport
  y : Inport  Port=2
  Calc Carry : Logic  AllPortsSameDT=off  OutDataTypeStr=boolean
  Calc Sum : Logic  Operator=XOR  AllPortsSameDT=off  OutDataTypeStr=boolean
  Sum : Outport
  Carry : Outport  Port=2
  wires:
  Calc Carry/1 -> Carry/1
  x/1 -> Calc Carry/1, Calc Sum/1
  Calc Sum/1 -> Sum/1
  y/1 -> Calc Sum/2, Calc Carry/2

== system labFinal_8/8-Bit_Processor/8-bit Multiply/2^36/Half_Adder1 ==
  x : Inport
  y : Inport  Port=2
  Calc Carry : Logic  AllPortsSameDT=off  OutDataTypeStr=boolean
  Calc Sum : Logic  Operator=XOR  AllPortsSameDT=off  OutDataTypeStr=boolean
  Sum : Outport
  Carry : Outport  Port=2
  wires:
  Calc Carry/1 -> Carry/1
  x/1 -> Calc Carry/1, Calc Sum/1
  Calc Sum/1 -> Sum/1
  y/1 -> Calc Sum/2, Calc Carry/2

== system labFinal_8/8-Bit_Processor/8-bit Multiply/2^37/Half_Adder ==
  x : Inport
  y : Inport  Port=2
  Calc Carry : Logic  AllPortsSameDT=off  OutDataTypeStr=boolean
  Calc Sum : Logic  Operator=XOR  AllPortsSameDT=off  OutDataTypeStr=boolean
  Sum : Outport
  Carry : Outport  Port=2
  wires:
  Calc Carry/1 -> Carry/1
  x/1 -> Calc Carry/1, Calc Sum/1
  Calc Sum/1 -> Sum/1
  y/1 -> Calc Sum/2, Calc Carry/2

== system labFinal_8/8-Bit_Processor/8-bit Multiply/2^37/Half_Adder1 ==
  x : Inport
  y : Inport  Port=2
  Calc Carry : Logic  AllPortsSameDT=off  OutDataTypeStr=boolean
  Calc Sum : Logic  Operator=XOR  AllPortsSameDT=off  OutDataTypeStr=boolean
  Sum : Outport
  Carry : Outport  Port=2
  wires:
  Calc Carry/1 -> Carry/1
  x/1 -> Calc Carry/1, Calc Sum/1
  Calc Sum/1 -> Sum/1
  y/1 -> Calc Sum/2, Calc Carry/2

== system labFinal_8/8-Bit_Processor/8-bit Multiply/2^38/Half_Adder ==
  x : Inport
  y : Inport  Port=2
  Calc Carry : Logic  AllPortsSameDT=off  OutDataTypeStr=boolean
  Calc Sum : Logic  Operator=XOR  AllPortsSameDT=off  OutDataTypeStr=boolean
  Sum : Outport
  Carry : Outport  Port=2
  wires:
  Calc Carry/1 -> Carry/1
  x/1 -> Calc Carry/1, Calc Sum/1
  Calc Sum/1 -> Sum/1
  y/1 -> Calc Sum/2, Calc Carry/2

== system labFinal_8/8-Bit_Processor/8-bit Multiply/2^38/Half_Adder1 ==
  x : Inport
  y : Inport  Port=2
  Calc Carry : Logic  AllPortsSameDT=off  OutDataTypeStr=boolean
  Calc Sum : Logic  Operator=XOR  AllPortsSameDT=off  OutDataTypeStr=boolean
  Sum : Outport
  Carry : Outport  Port=2
  wires:
  Calc Carry/1 -> Carry/1
  x/1 -> Calc Carry/1, Calc Sum/1
  Calc Sum/1 -> Sum/1
  y/1 -> Calc Sum/2, Calc Carry/2

== system labFinal_8/8-Bit_Processor/8-bit Multiply/2^39/Half_Adder ==
  x : Inport
  y : Inport  Port=2
  Calc Carry : Logic  AllPortsSameDT=off  OutDataTypeStr=boolean
  Calc Sum : Logic  Operator=XOR  AllPortsSameDT=off  OutDataTypeStr=boolean
  Sum : Outport
  Carry : Outport  Port=2
  wires:
  Calc Carry/1 -> Carry/1
  x/1 -> Calc Carry/1, Calc Sum/1
  Calc Sum/1 -> Sum/1
  y/1 -> Calc Sum/2, Calc Carry/2

== system labFinal_8/8-Bit_Processor/8-bit Multiply/2^39/Half_Adder1 ==
  x : Inport
  y : Inport  Port=2
  Calc Carry : Logic  AllPortsSameDT=off  OutDataTypeStr=boolean
  Calc Sum : Logic  Operator=XOR  AllPortsSameDT=off  OutDataTypeStr=boolean
  Sum : Outport
  Carry : Outport  Port=2
  wires:
  Calc Carry/1 -> Carry/1
  x/1 -> Calc Carry/1, Calc Sum/1
  Calc Sum/1 -> Sum/1
  y/1 -> Calc Sum/2, Calc Carry/2

== system labFinal_8/8-Bit_Processor/8-bit Multiply/2^4/Half_Adder ==
  x : Inport
  y : Inport  Port=2
  Calc Carry : Logic  AllPortsSameDT=off  OutDataTypeStr=boolean
  Calc Sum : Logic  Operator=XOR  AllPortsSameDT=off  OutDataTypeStr=boolean
  Sum : Outport
  Carry : Outport  Port=2
  wires:
  Calc Carry/1 -> Carry/1
  x/1 -> Calc Carry/1, Calc Sum/1
  Calc Sum/1 -> Sum/1
  y/1 -> Calc Sum/2, Calc Carry/2

== system labFinal_8/8-Bit_Processor/8-bit Multiply/2^4/Half_Adder1 ==
  x : Inport
  y : Inport  Port=2
  Calc Carry : Logic  AllPortsSameDT=off  OutDataTypeStr=boolean
  Calc Sum : Logic  Operator=XOR  AllPortsSameDT=off  OutDataTypeStr=boolean
  Sum : Outport
  Carry : Outport  Port=2
  wires:
  Calc Carry/1 -> Carry/1
  x/1 -> Calc Carry/1, Calc Sum/1
  Calc Sum/1 -> Sum/1
  y/1 -> Calc Sum/2, Calc Carry/2

== system labFinal_8/8-Bit_Processor/8-bit Multiply/2^5/Half_Adder ==
  x : Inport
  y : Inport  Port=2
  Calc Carry : Logic  AllPortsSameDT=off  OutDataTypeStr=boolean
  Calc Sum : Logic  Operator=XOR  AllPortsSameDT=off  OutDataTypeStr=boolean
  Sum : Outport
  Carry : Outport  Port=2
  wires:
  Calc Carry/1 -> Carry/1
  x/1 -> Calc Carry/1, Calc Sum/1
  Calc Sum/1 -> Sum/1
  y/1 -> Calc Sum/2, Calc Carry/2

== system labFinal_8/8-Bit_Processor/8-bit Multiply/2^5/Half_Adder1 ==
  x : Inport
  y : Inport  Port=2
  Calc Carry : Logic  AllPortsSameDT=off  OutDataTypeStr=boolean
  Calc Sum : Logic  Operator=XOR  AllPortsSameDT=off  OutDataTypeStr=boolean
  Sum : Outport
  Carry : Outport  Port=2
  wires:
  Calc Carry/1 -> Carry/1
  x/1 -> Calc Carry/1, Calc Sum/1
  Calc Sum/1 -> Sum/1
  y/1 -> Calc Sum/2, Calc Carry/2

== system labFinal_8/8-Bit_Processor/8-bit Multiply/2^6/Half_Adder ==
  x : Inport
  y : Inport  Port=2
  Calc Carry : Logic  AllPortsSameDT=off  OutDataTypeStr=boolean
  Calc Sum : Logic  Operator=XOR  AllPortsSameDT=off  OutDataTypeStr=boolean
  Sum : Outport
  Carry : Outport  Port=2
  wires:
  Calc Carry/1 -> Carry/1
  x/1 -> Calc Carry/1, Calc Sum/1
  Calc Sum/1 -> Sum/1
  y/1 -> Calc Sum/2, Calc Carry/2

== system labFinal_8/8-Bit_Processor/8-bit Multiply/2^6/Half_Adder1 ==
  x : Inport
  y : Inport  Port=2
  Calc Carry : Logic  AllPortsSameDT=off  OutDataTypeStr=boolean
  Calc Sum : Logic  Operator=XOR  AllPortsSameDT=off  OutDataTypeStr=boolean
  Sum : Outport
  Carry : Outport  Port=2
  wires:
  Calc Carry/1 -> Carry/1
  x/1 -> Calc Carry/1, Calc Sum/1
  Calc Sum/1 -> Sum/1
  y/1 -> Calc Sum/2, Calc Carry/2

== system labFinal_8/8-Bit_Processor/8-bit Multiply/2^7/Half_Adder ==
  x : Inport
  y : Inport  Port=2
  Calc Carry : Logic  AllPortsSameDT=off  OutDataTypeStr=boolean
  Calc Sum : Logic  Operator=XOR  AllPortsSameDT=off  OutDataTypeStr=boolean
  Sum : Outport
  Carry : Outport  Port=2
  wires:
  Calc Carry/1 -> Carry/1
  x/1 -> Calc Carry/1, Calc Sum/1
  Calc Sum/1 -> Sum/1
  y/1 -> Calc Sum/2, Calc Carry/2

== system labFinal_8/8-Bit_Processor/8-bit Multiply/2^7/Half_Adder1 ==
  x : Inport
  y : Inport  Port=2
  Calc Carry : Logic  AllPortsSameDT=off  OutDataTypeStr=boolean
  Calc Sum : Logic  Operator=XOR  AllPortsSameDT=off  OutDataTypeStr=boolean
  Sum : Outport
  Carry : Outport  Port=2
  wires:
  Calc Carry/1 -> Carry/1
  x/1 -> Calc Carry/1, Calc Sum/1
  Calc Sum/1 -> Sum/1
  y/1 -> Calc Sum/2, Calc Carry/2

== system labFinal_8/8-Bit_Processor/8-bit Multiply/2^9/Half_Adder ==
  x : Inport
  y : Inport  Port=2
  Calc Carry : Logic  AllPortsSameDT=off  OutDataTypeStr=boolean
  Calc Sum : Logic  Operator=XOR  AllPortsSameDT=off  OutDataTypeStr=boolean
  Sum : Outport
  Carry : Outport  Port=2
  wires:
  Calc Carry/1 -> Carry/1
  x/1 -> Calc Carry/1, Calc Sum/1
  Calc Sum/1 -> Sum/1
  y/1 -> Calc Sum/2, Calc Carry/2

== system labFinal_8/8-Bit_Processor/8-bit Multiply/2^9/Half_Adder1 ==
  x : Inport
  y : Inport  Port=2
  Calc Carry : Logic  AllPortsSameDT=off  OutDataTypeStr=boolean
  Calc Sum : Logic  Operator=XOR  AllPortsSameDT=off  OutDataTypeStr=boolean
  Sum : Outport
  Carry : Outport  Port=2
  wires:
  Calc Carry/1 -> Carry/1
  x/1 -> Calc Carry/1, Calc Sum/1
  Calc Sum/1 -> Sum/1
  y/1 -> Calc Sum/2, Calc Carry/2

== system labFinal_8/8-Bit_Processor/8-bit Multiply/Subsystem/Slicer A ==
  uint8 : Inport  OutDataTypeStr=uint8  SampleTime=1
  Bit Slice : hdlsllib/Logic and Bit Operations/Bit Slice  lidx=0  ridx=0
  Bit Slice1 : hdlsllib/Logic and Bit Operations/Bit Slice  lidx=1  ridx=1
  Bit Slice2 : hdlsllib/Logic and Bit Operations/Bit Slice  lidx=2  ridx=2
  Bit Slice3 : hdlsllib/Logic and Bit Operations/Bit Slice  lidx=3  ridx=3
  Bit Slice4 : hdlsllib/Logic and Bit Operations/Bit Slice  lidx=4  ridx=4
  Bit Slice5 : hdlsllib/Logic and Bit Operations/Bit Slice  lidx=5  ridx=5
  Bit Slice6 : hdlsllib/Logic and Bit Operations/Bit Slice  lidx=6  ridx=6
  Bit Slice7 : hdlsllib/Logic and Bit Operations/Bit Slice  lidx=7  ridx=7
  Data Type Conversion{,1..7} (8 alike) : DataTypeConversion  OutDataTypeStr=boolean
  A 2^7 : Outport
  A 2^6 : Outport  Port=2
  A 2^5 : Outport  Port=3
  A 2^4 : Outport  Port=4
  A 2^3 : Outport  Port=5
  A 2^2 : Outport  Port=6
  A 2^1 : Outport  Port=7
  "A 2^0 " : Outport  Port=8
  wires:
  Data Type Conversion/1 -> "A 2^0 "/1
  Data Type Conversion5/1 -> A 2^5/1
  Bit Slice1/1 -> Data Type Conversion1/1
  Bit Slice5/1 -> Data Type Conversion5/1
  Bit Slice7/1 -> Data Type Conversion7/1
  Bit Slice2/1 -> Data Type Conversion2/1
  Bit Slice3/1 -> Data Type Conversion3/1
  Data Type Conversion6/1 -> A 2^6/1
  Bit Slice4/1 -> Data Type Conversion4/1
  uint8/1 -> Bit Slice4/1, Bit Slice5/1, Bit Slice6/1, Bit Slice7/1, Bit Slice3/1, Bit Slice2/1, Bit Slice1/1, Bit Slice/1
  Data Type Conversion1/1 -> A 2^1/1
  Data Type Conversion2/1 -> A 2^2/1
  Bit Slice/1 -> Data Type Conversion/1
  Bit Slice6/1 -> Data Type Conversion6/1
  Data Type Conversion3/1 -> A 2^3/1
  Data Type Conversion4/1 -> A 2^4/1
  Data Type Conversion7/1 -> A 2^7/1

== system labFinal_8/8-Bit_Processor/8-bit Multiply/Subsystem/Slicer B ==
  uint8 : Inport  OutDataTypeStr=uint8  SampleTime=1
  Bit Slice : hdlsllib/Logic and Bit Operations/Bit Slice  lidx=0  ridx=0
  Bit Slice1 : hdlsllib/Logic and Bit Operations/Bit Slice  lidx=1  ridx=1
  Bit Slice2 : hdlsllib/Logic and Bit Operations/Bit Slice  lidx=2  ridx=2
  Bit Slice3 : hdlsllib/Logic and Bit Operations/Bit Slice  lidx=3  ridx=3
  Bit Slice4 : hdlsllib/Logic and Bit Operations/Bit Slice  lidx=4  ridx=4
  Bit Slice5 : hdlsllib/Logic and Bit Operations/Bit Slice  lidx=5  ridx=5
  Bit Slice6 : hdlsllib/Logic and Bit Operations/Bit Slice  lidx=6  ridx=6
  Bit Slice7 : hdlsllib/Logic and Bit Operations/Bit Slice  lidx=7  ridx=7
  Data Type Conversion{,1..7} (8 alike) : DataTypeConversion  OutDataTypeStr=boolean
  "B 2^0 " : Outport
  B 2^1 : Outport  Port=2
  B 2^2 : Outport  Port=3
  B 2^3 : Outport  Port=4
  B 2^4 : Outport  Port=5
  B 2^5 : Outport  Port=6
  B 2^6 : Outport  Port=7
  B 2^7 : Outport  Port=8
  wires:
  Data Type Conversion/1 -> "B 2^0 "/1
  Data Type Conversion5/1 -> B 2^5/1
  Bit Slice1/1 -> Data Type Conversion1/1
  Bit Slice5/1 -> Data Type Conversion5/1
  Bit Slice7/1 -> Data Type Conversion7/1
  Bit Slice2/1 -> Data Type Conversion2/1
  Bit Slice3/1 -> Data Type Conversion3/1
  Data Type Conversion6/1 -> B 2^6/1
  Bit Slice4/1 -> Data Type Conversion4/1
  uint8/1 -> Bit Slice4/1, Bit Slice5/1, Bit Slice6/1, Bit Slice7/1, Bit Slice3/1, Bit Slice2/1, Bit Slice1/1, Bit Slice/1
  Data Type Conversion1/1 -> B 2^1/1
  Data Type Conversion2/1 -> B 2^2/1
  Bit Slice/1 -> Data Type Conversion/1
  Bit Slice6/1 -> Data Type Conversion6/1
  Data Type Conversion3/1 -> B 2^3/1
  Data Type Conversion4/1 -> B 2^4/1
  Data Type Conversion7/1 -> B 2^7/1

== system labFinal_8/8-Bit_Processor/8-bit Subtractor/2^0/Half_Adder ==
  x : Inport
  y : Inport  Port=2
  Calc Carry : Logic  AllPortsSameDT=off  OutDataTypeStr=boolean
  Calc Sum : Logic  Operator=XOR  AllPortsSameDT=off  OutDataTypeStr=boolean
  Sum : Outport
  Carry : Outport  Port=2
  wires:
  Calc Carry/1 -> Carry/1
  x/1 -> Calc Carry/1, Calc Sum/1
  Calc Sum/1 -> Sum/1
  y/1 -> Calc Sum/2, Calc Carry/2
